simulink model "AnalogBilinearParaEq"  (R2018b)
settings: Solver=FixedStepAuto  StartTime=0.0  StopTime=inf  RelTol=1e-3  EnableMultiTasking=on
values from neighbouring files (symbols this model uses):
  AAnalog = AAnalog'    [ParaEq_5Tab.m]
  BAnalog = BAnalog'    [ParaEq_5Tab.m]
libraries: stm32f769ilib x2, dsparch4 x1
settings Model: SimulationMode=external  Creator=hpong  LastModifiedBy=hpong
settings OptimizationCC: EnhancedBackFolding=on  PassReuseOutputArgsAs=Individual arguments  MaxStackSize=64  OptimizeBlockOrder=speed  DifferentSizesBufferReuse=on  OptimizationCustomize=off
settings DebuggingCC: ParameterTunabilityLossMsg=error  LibraryContextMissingDiagnostic=none
settings HardwareCC: ProdBitPerPointer=32  ProdBitPerSizeT=32  ProdBitPerPtrDiffT=32  ProdLargestAtomicInteger=Long  ProdLargestAtomicFloat=Double  ProdWordSize=32  ProdHWDeviceType=ARM Compatible->ARM Cortex
settings SFSimCC: SimUseLocalCustomCode=off  MATLABDynamicMemAlloc=off
settings RTWCC: SystemTargetFile=ert.tlc  HardwareBoard=STM32F769I-Discovery  TemplateMakefile=ert_default_tmf  GenerateReport=on  RTWUseLocalCustomCode=off  Toolchain=GNU Tools for ARM Embedded Processors  IncludeHyperlinkInReport=on  LaunchReport=on  GenerateTraceInfo=on  GenerateTraceReport=on  GenerateTraceReportSl=on  GenerateTraceReportSf=on  GenerateTraceReportEml=on
settings CodeAppCC: ForceParamTrailComments=on  IgnoreCustomStorageClasses=off  OperatorAnnotations=on  SimulinkDataObjDesc=on  SFDataObjDesc=on  InsertBlockDesc=on
settings ERTTargetCC: CodeReplacementLibrary=ARM Cortex-M (CMSIS)

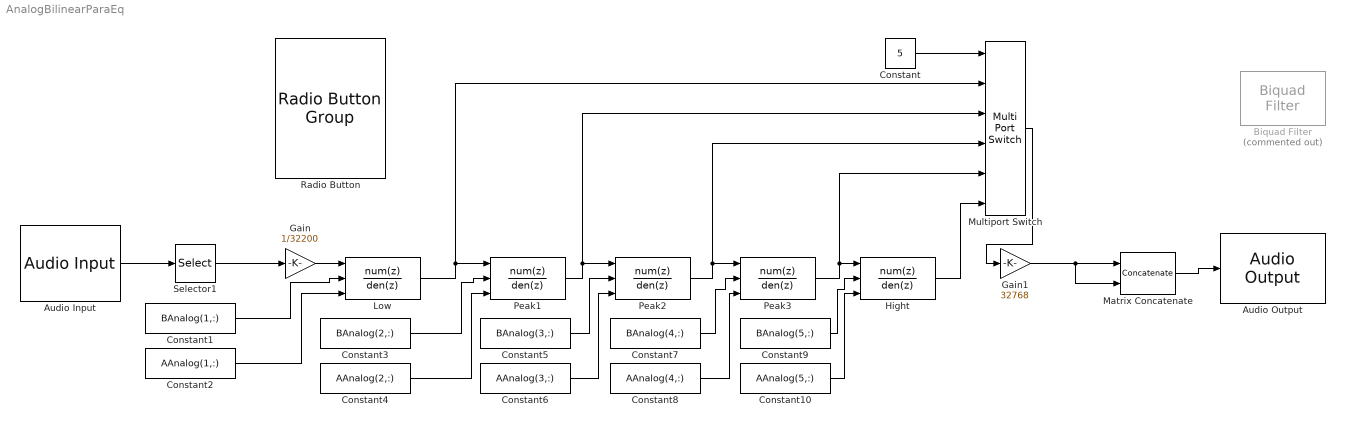
== system AnalogBilinearParaEq ==
  Audio Input : stm32f769ilib/Audio Input  InputDevice=LineIn  SamplingFreq=44100  NumCh=2  FrameSize=100
      settings: SourceProductName=Embedded Coder Support Package for STMicroelectronics Discovery Boards  SourceProductBaseCode=STMICRODIS
  Audio Output : stm32f769ilib/Audio Output  OutputDevice=Headphone  SamplingFreq=44100  Volume=63
      settings: SourceProductName=Embedded Coder Support Package for STMicroelectronics Discovery Boards  SourceProductBaseCode=STMICRODIS
  Biquad Filter : dsparch4/Biquad Filter  Commented=on  FilterSource=Dialog parameters  CoeffSource=Specify via dialog  FilterObject=BQF  IIRFiltStruct=Direct form II transposed  BiQuadCoeffs=|  ScaleValues=1  IC=0  ICnum=0  ICden=0  a0Flag=Warning  optimizeScaleValues=on  ScaleValueMode=Specify via input port (g)  InputProcessing=Columns as channels (frame based)  roundingMode=Floor  overflowMode=off  scaleValueFracLength=14  denProdOutputFracLength=30  denAccumFracLength=30  secondMemoryFracLength=15
      | [1.00285240153205	-1.96968575141370	0.967468878543926	1	-1.96977855582618	0.970228475663498
      | 0.978903241987940	-1.90050214129549	0.924689401200335	1	-1.90050214129549	0.903592643188274
      | 1.03027325119350	-1.95201740751769	0.941725487219076	1	-1.95201740751769	0.971998738412580
      | 0.962747894922692	-1.57170990847482	0.675003985824103	1	-1.57170990847482	0.637751880746795
      | 0.714507945856894	-0.122353334089159	0.126297400311252	1	-0.497156618811420	0.215608630890407]
      settings: SourceProductName=DSP System Toolbox
  Constant : Constant  Value=5
  Constant1 : Constant  Value=BAnalog(1,:)
  Constant10 : Constant  Value=AAnalog(5,:)
  Constant2 : Constant  Value=AAnalog(1,:)
  Constant3 : Constant  Value=BAnalog(2,:)
  Constant4 : Constant  Value=AAnalog(2,:)
  Constant5 : Constant  Value=BAnalog(3,:)
  Constant6 : Constant  Value=AAnalog(3,:)
  Constant7 : Constant  Value=BAnalog(4,:)
  Constant8 : Constant  Value=AAnalog(4,:)
  Constant9 : Constant  Value=BAnalog(5,:)
  Gain : Gain  Gain=1/32200  OutDataTypeStr=double
  Gain1 : Gain  Gain=32768  OutDataTypeStr=int16
  Hight : DiscreteFilter  NumeratorSource=Input port  Numerator="[0.714507945856894\t-0.122353334089159\t0.126297400311252]"  DenominatorSource=Input port  Denominator=[1,-0.497156618811420,0.215608630890407]  InitialStates=1  InputProcessing=Columns as channels (frame based)  a0EqualsOne=on
      settings: InputPortMap=u0,p1,p3
  Low : DiscreteFilter  NumeratorSource=Input port  Numerator="[1.00285240153205\t-1.96968575141370\t0.967468878543926]"  DenominatorSource=Input port  Denominator="[1\t-1.96977855582618\t0.970228475663498]"  InitialStates=1  InputProcessing=Columns as channels (frame based)  a0EqualsOne=on
      settings: InputPortMap=u0,p1,p3
  Matrix Concatenate : Concatenate  Mode=Multidimensional array  ConcatenateDimension=2
  Multiport Switch : MultiPortSwitch  Inputs=5
  Peak1 : DiscreteFilter  NumeratorSource=Input port  Numerator=[0.978903241987940,-1.90050214129549,0.924689401200335]  DenominatorSource=Input port  Denominator=[1,-1.90050214129549,0.903592643188274]  InitialStates=1  InputProcessing=Columns as channels (frame based)  a0EqualsOne=on
      settings: InputPortMap=u0,p1,p3
  Peak2 : DiscreteFilter  NumeratorSource=Input port  Numerator=[1.03027325119350,-1.95201740751769,0.941725487219076]  DenominatorSource=Input port  Denominator=[1,-1.95201740751769,0.971998738412580]  InitialStates=1  InputProcessing=Columns as channels (frame based)  a0EqualsOne=on
      settings: InputPortMap=u0,p1,p3
  Peak3 : DiscreteFilter  NumeratorSource=Input port  Numerator=[0.962747894922692,-1.57170990847482,0.675003985824103]  DenominatorSource=Input port  Denominator=[1,-1.57170990847482,0.637751880746795]  InitialStates=1  InputProcessing=Columns as channels (frame based)  a0EqualsOne=on
      settings: InputPortMap=u0,p1,p3
  Radio Button : RadioButtonGroup  WebBlockId=70  SelectedLabel=LP Shelving  ButtonGroupName=Group
      settings: Values={{'HP Shelving', 'Peak3', 'Peak2', 'Peak1', 'LP Shelving'}, [1 2 3 4 5]}
  Selector1 : Selector  NumberOfDimensions=2  InputPortWidth=2  IndexOptions=Select all,Index vector (dialog)  Indices=1,1  OutputSizes=1,1
  wires:
  Matrix Concatenate/1 -> Audio Output/1
  Audio Input/1 -> Selector1/1
  Selector1/1 -> Gain/1
  Gain1/1 -> Matrix Concatenate/2, Matrix Concatenate/1
  Peak1/1 -> Multiport Switch/3, Peak2/1
  Low/1 -> Multiport Switch/2, Peak1/1
  Peak2/1 -> Multiport Switch/4, Peak3/1
  Peak3/1 -> Multiport Switch/5, Hight/1
  Multiport Switch/1 -> Gain1/1
  Gain/1 -> Low/1
  Constant/1 -> Multiport Switch/1
  Constant1/1 -> Low/2
  Constant2/1 -> Low/3
  Hight/1 -> Multiport Switch/6
  Constant3/1 -> Peak1/2
  Constant4/1 -> Peak1/3
  Constant5/1 -> Peak2/2
  Constant6/1 -> Peak2/3
  Constant8/1 -> Peak3/3
  Constant7/1 -> Peak3/2
  Constant10/1 -> Hight/3
  Constant9/1 -> Hight/2
